simulink model "duplicateTest_after"  (R2017a)
settings: Solver=VariableStepAuto  StartTime=0.0  StopTime=10.0  RelTol=1e-3
settings Model: Creator=GM  LastModifiedBy=GM

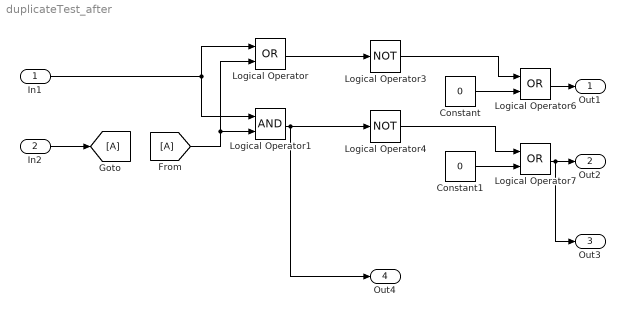
== system duplicateTest_after ==
  In1 : Inport
  In2 : Inport  Port=2
  Constant : Constant  Value=0
  Constant1 : Constant  Value=0
  Logical Operator : Logic  Operator=OR  AllPortsSameDT=off  OutDataTypeStr=boolean
  Logical Operator1 : Logic  AllPortsSameDT=off  OutDataTypeStr=boolean
  Logical Operator3 : Logic  Operator=NOT  AllPortsSameDT=off  OutDataTypeStr=boolean
  Logical Operator4 : Logic  Operator=NOT  AllPortsSameDT=off  OutDataTypeStr=boolean
  Logical Operator6 : Logic  Operator=OR  AllPortsSameDT=off  OutDataTypeStr=boolean
  Logical Operator7 : Logic  Operator=OR  AllPortsSameDT=off  OutDataTypeStr=boolean
  Out1 : Outport
  Out2 : Outport  Port=2
  Out3 : Outport  Port=3
  Out4 : Outport  Port=4
  wires:
  In2/1 -> [A]
  In1/1 -> Logical Operator/1, Logical Operator1/1
  [A] -> Logical Operator1/2, Logical Operator/2
  Logical Operator/1 -> Logical Operator3/1
  Logical Operator1/1 -> Logical Operator4/1, Out4/1
  Constant/1 -> Logical Operator6/2
  Constant1/1 -> Logical Operator7/2
  Logical Operator4/1 -> Logical Operator7/1
  Logical Operator3/1 -> Logical Operator6/1
  Logical Operator6/1 -> Out1/1
  Logical Operator7/1 -> Out2/1, Out3/1
